simulink model "Cw1_Sim_Fcn"  (R2014a)
settings: Solver=ode45  StartTime=0.0  StopTime=0.02  RelTol=1e-3
values from neighbouring files (symbols this model uses):
  omega = 2*pi*f    (= 314.159265359)    [Scw1_Simulink.m]
  Um = UN*2^0.5    (= 325.269119346)    [Scw1_Simulink.m]
  UN = 230    [Scw1_Simulink.m]
libraries: simulink x1
settings Model: Creator=user  LastModifiedBy=user

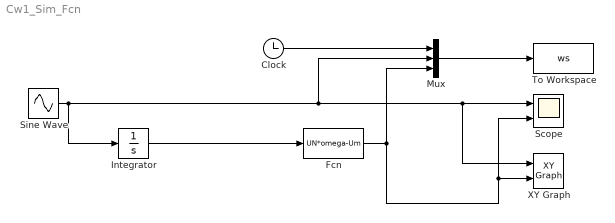
== system Cw1_Sim_Fcn ==
  Clock : Clock
  Fcn : Fcn  Expr=UN*omega-Um
  Integrator : Integrator
  Mux : Mux  Inputs=3
  Scope : Scope  NumInputPorts=2
      settings: YMin=-5~-5  YMax=5~5
  Sine Wave : Sin  Amplitude=230*2^0.5  Frequency=2*pi*50  SampleTime=0
  To Workspace : ToWorkspace  VariableName=ws  SampleTime=-1
  XY Graph : simulink/Sinks/XY Graph  xmin=-500  xmax=500  ymin=-500  ymax=500  st=-1
  wires:
  Sine Wave/1 -> Integrator/1, Mux/2, XY Graph/1, Scope/1
  Fcn/1 -> XY Graph/2, Scope/2, Mux/3
  Clock/1 -> Mux/1
  Mux/1 -> To Workspace/1
  Integrator/1 -> Fcn/1
